simulink library "Surface_Profile_Axle3_None"  (R2025b)
settings: Solver=VariableStepAuto  StartTime=0.0  StopTime=10.0  RelTol=1e-3
Description:
  | Simscape Vehicle Templates Library
  | 
  | Copyright 2018-2025 The MathWorks, Inc.
settings Model: Creator=smiller  LastModifiedBy=smiller
settings ModelReferenceCC: EnableRefExpFcnMdlSchedulingChecks=on
settings RTWCC: GPUComputeCapability=3.5

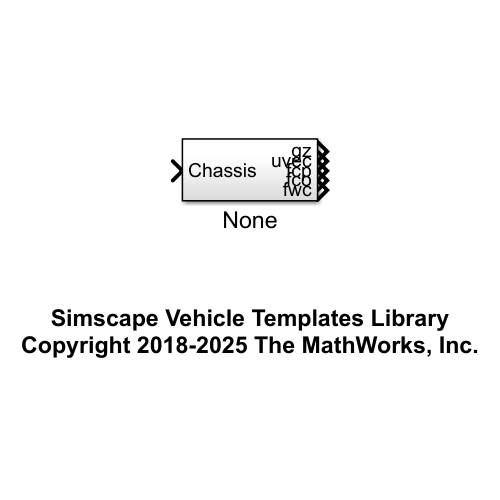
[thumbnail: Simulink's stored preview of the top-level diagram]
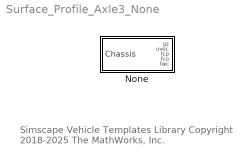
== system Surface_Profile_Axle3_None ==
  note: Simscape Vehicle Templates Library
      | Copyright 2018-2025 The MathWorks, Inc.
  None : Subsystem  VariantControl=None

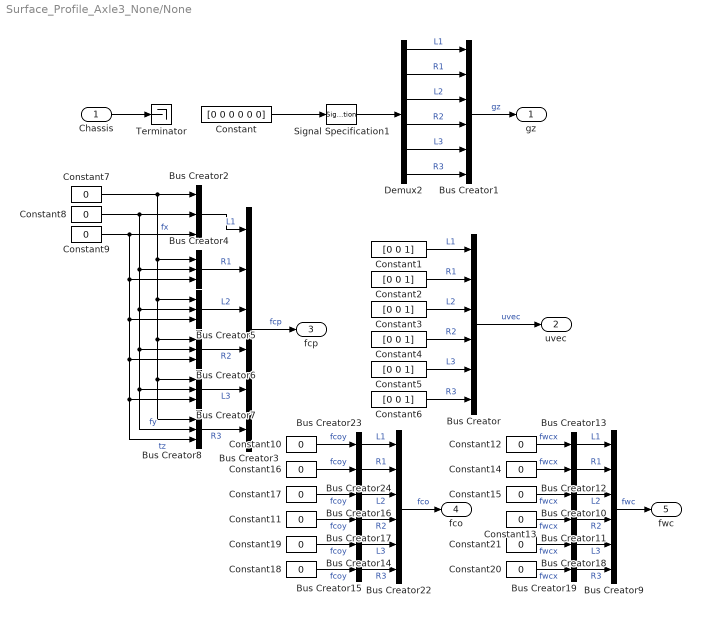
== system Surface_Profile_Axle3_None/None ==
  Chassis : Inport
  Bus Creator{,1,3,9,22} (5 alike) : BusCreator  Inputs=6
  Bus Creator{10..19,23..24} (12 alike) : BusCreator  Inputs=1
  Bus Creator{2,4..8} (6 alike) : BusCreator  Inputs=3
  Constant : Constant  Value=[0 0 0 0 0 0]
  Constant{1..6} (6 alike) : Constant  Value=[0 0 1]
  Constant{7..21} (15 alike) : Constant  Value=0
  Demux2 : Demux  Outputs=6
  Signal Specification1 : SignalSpecification  Unit=m
  Terminator : Terminator
  gz : Outport  VectorParamsAs1DForOutWhenUnconnected=off
  uvec : Outport  Port=2  VectorParamsAs1DForOutWhenUnconnected=off
  fcp : Outport  Port=3  VectorParamsAs1DForOutWhenUnconnected=off
  fco : Outport  Port=4  VectorParamsAs1DForOutWhenUnconnected=off
  fwc : Outport  Port=5  VectorParamsAs1DForOutWhenUnconnected=off
  wires:
  Constant5/1 -> Bus Creator/5  "L3"
  Constant6/1 -> Bus Creator/6  "R3"
  Demux2/6 -> Bus Creator1/6  "R3"
  Demux2/5 -> Bus Creator1/5  "L3"
  Chassis/1 -> Terminator/1
  Constant/1 -> Signal Specification1/1
  Demux2/1 -> Bus Creator1/1  "L1"
  Signal Specification1/1 -> Demux2/1
  Bus Creator1/1 -> gz/1  "gz"
  Demux2/2 -> Bus Creator1/2  "R1"
  Demux2/4 -> Bus Creator1/4  "R2"
  Demux2/3 -> Bus Creator1/3  "L2"
  Constant3/1 -> Bus Creator/3  "L2"
  Constant2/1 -> Bus Creator/2  "R1"
  Constant1/1 -> Bus Creator/1  "L1"
  Constant4/1 -> Bus Creator/4  "R2"
  Bus Creator/1 -> uvec/1  "uvec"
  Bus Creator6/1 -> Bus Creator3/4  "R2"
  Bus Creator5/1 -> Bus Creator3/3  "L2"
  Bus Creator4/1 -> Bus Creator3/2  "R1"
  Bus Creator2/1 -> Bus Creator3/1  "L1"
  Bus Creator3/1 -> fcp/1  "fcp"
  Bus Creator7/1 -> Bus Creator3/5  "L3"
  Bus Creator8/1 -> Bus Creator3/6  "R3"
  Constant9/1 -> Bus Creator2/3, Bus Creator4/3, Bus Creator5/3, Bus Creator6/3, Bus Creator7/3, Bus Creator8/3  "tz"
  Constant8/1 -> Bus Creator2/2, Bus Creator4/2, Bus Creator5/2, Bus Creator6/2, Bus Creator7/2, Bus Creator8/2  "fy"
  Constant7/1 -> Bus Creator2/1, Bus Creator4/1, Bus Creator5/1, Bus Creator8/1, Bus Creator7/1, Bus Creator6/1  "fx"
  Constant21/1 -> Bus Creator18/1  "fwcx"
  Constant14/1 -> Bus Creator12/1  "fwcx"
  Constant16/1 -> Bus Creator24/1  "fcoy"
  Bus Creator10/1 -> Bus Creator9/3  "L2"
  Constant11/1 -> Bus Creator17/1  "fcoy"
  Bus Creator13/1 -> Bus Creator9/1  "L1"
  Bus Creator23/1 -> Bus Creator22/1  "L1"
  Bus Creator17/1 -> Bus Creator22/4  "R2"
  Constant15/1 -> Bus Creator10/1  "fwcx"
  Bus Creator22/1 -> fco/1  "fco"
  Constant18/1 -> Bus Creator15/1  "fcoy"
  Bus Creator15/1 -> Bus Creator22/6  "R3"
  Bus Creator14/1 -> Bus Creator22/5  "L3"
  Bus Creator18/1 -> Bus Creator9/5  "L3"
  Constant13/1 -> Bus Creator11/1  "fwcx"
  Bus Creator9/1 -> fwc/1  "fwc"
  Constant19/1 -> Bus Creator14/1  "fcoy"
  Bus Creator19/1 -> Bus Creator9/6  "R3"
  Bus Creator24/1 -> Bus Creator22/2  "R1"
  Constant17/1 -> Bus Creator16/1  "fcoy"
  Bus Creator16/1 -> Bus Creator22/3  "L2"
  Constant20/1 -> Bus Creator19/1  "fwcx"
  Constant12/1 -> Bus Creator13/1  "fwcx"
  Constant10/1 -> Bus Creator23/1  "fcoy"
  Bus Creator12/1 -> Bus Creator9/2  "R1"
  Bus Creator11/1 -> Bus Creator9/4  "R2"
